simulink model "lab1_product_gain"  (R2019a)
settings: Solver=VariableStepAuto  StartTime=0.0  StopTime=10.0  RelTol=1e-3
settings Model: Creator=LEGION  LastModifiedBy=LEGION

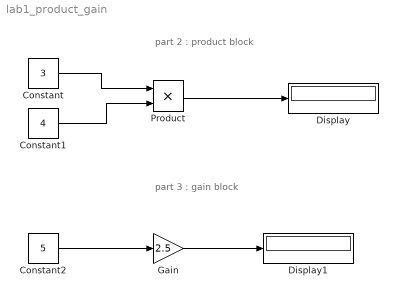
== system lab1_product_gain ==
  note: part 3 : gain block
  note: part 2 : product block
  Constant : Constant  Value=3
  Constant1 : Constant  Value=4
  Constant2 : Constant  Value=5
  Display : Display
  Display1 : Display
  Gain : Gain  Gain=2.5
  Product : Product
  wires:
  Constant/1 -> Product/1
  Constant1/1 -> Product/2
  Product/1 -> Display/1
  Constant2/1 -> Gain/1
  Gain/1 -> Display1/1
